simulink model "APP_Coherency_System_Rev_0"  (R2022b)
settings: Solver=VariableStepAuto  StartTime=0.0  StopTime=1  MaxStep=1e-3  RelTol=1e-3
libraries: simulink x2
settings Model: Creator=HiTech  LastModifiedBy=HiTech

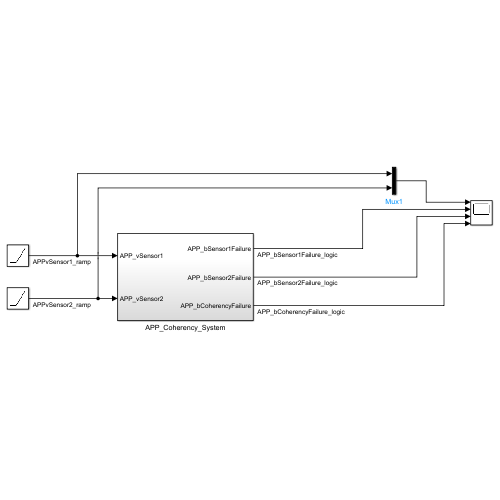
[thumbnail: Simulink's stored preview of the top-level diagram]
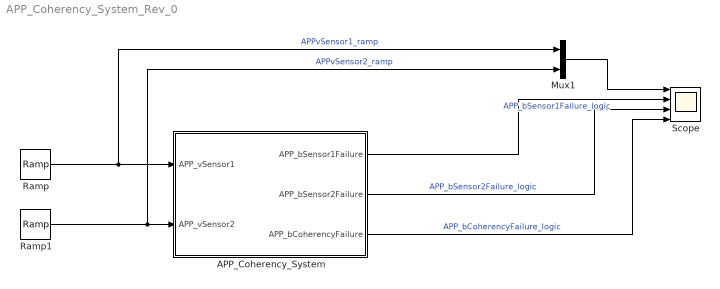
== system APP_Coherency_System_Rev_0 ==
  APP_Coherency_System : Subsystem
  Mux1 : Mux  Inputs=2
  Ramp : simulink/Sources/Ramp  slope=0  start=0  InitialOutput=0
  Ramp1 : simulink/Sources/Ramp  slope=-4  start=0  InitialOutput=4.5
  Scope : Scope  NumInputPorts=4
  wires:
  Ramp/1 -> Mux1/1, APP_Coherency_System/1(APP_vSensor1)  "APPvSensor1_ramp"
  Ramp1/1 -> Mux1/2, APP_Coherency_System/2(APP_vSensor2)  "APPvSensor2_ramp"
  Mux1/1 -> Scope/1
  APP_Coherency_System/1(APP_bSensor1Failure) -> Scope/2  "APP_bSensor1Failure_logic"
  APP_Coherency_System/2(APP_bSensor2Failure) -> Scope/3  "APP_bSensor2Failure_logic"
  APP_Coherency_System/3(APP_bCoherencyFailure) -> Scope/4  "APP_bCoherencyFailure_logic"

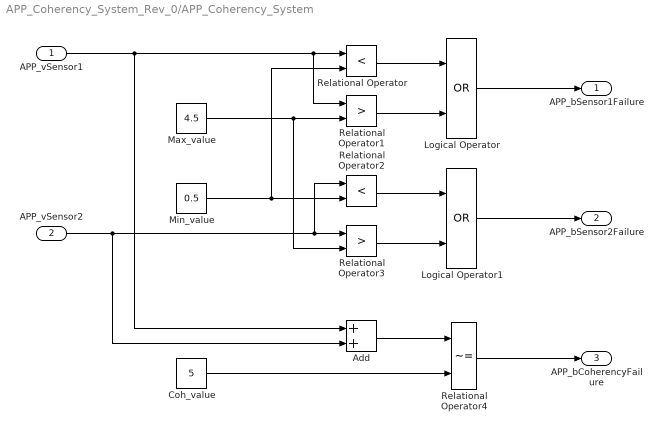
== system APP_Coherency_System_Rev_0/APP_Coherency_System ==
  APP_vSensor1 : Inport
  APP_vSensor2 : Inport  Port=2
  Add : Sum
  Coh_value : Constant  Value=5
  Logical Operator : Logic  Operator=OR  AllPortsSameDT=off  OutDataTypeStr=boolean
  Logical Operator1 : Logic  Operator=OR  AllPortsSameDT=off  OutDataTypeStr=boolean
  Max_value : Constant  Value=4.5
  Min_value : Constant  Value=0.5
  Relational Operator : RelationalOperator  Operator=<  OutDataTypeStr=boolean  RndMeth=Simplest  InputSameDT=off
  Relational Operator1 : RelationalOperator  Operator=>  OutDataTypeStr=boolean  RndMeth=Simplest  InputSameDT=off
  Relational Operator2 : RelationalOperator  Operator=<  OutDataTypeStr=boolean  RndMeth=Simplest  InputSameDT=off
  Relational Operator3 : RelationalOperator  Operator=>  OutDataTypeStr=boolean  RndMeth=Simplest  InputSameDT=off
  Relational Operator4 : RelationalOperator  Operator=~=  OutDataTypeStr=boolean  RndMeth=Simplest  InputSameDT=off
  APP_bSensor1Failure : Outport
  APP_bSensor2Failure : Outport  Port=2
  APP_bCoherencyFailure : Outport  Port=3
  wires:
  Logical Operator/1 -> APP_bSensor1Failure/1
  Relational Operator/1 -> Logical Operator/1
  Relational Operator1/1 -> Logical Operator/2
  Relational Operator3/1 -> Logical Operator1/2
  Relational Operator2/1 -> Logical Operator1/1
  Logical Operator1/1 -> APP_bSensor2Failure/1
  Relational Operator4/1 -> APP_bCoherencyFailure/1
  Min_value/1 -> Relational Operator/2, Relational Operator2/2
  Max_value/1 -> Relational Operator3/2, Relational Operator1/2
  APP_vSensor1/1 -> Add/1, Relational Operator1/1, Relational Operator/1
  APP_vSensor2/1 -> Add/2, Relational Operator2/1, Relational Operator3/1
  Add/1 -> Relational Operator4/1
  Coh_value/1 -> Relational Operator4/2
